simulink model "VCU_CS75_12_30_test"  (R2014a)
settings: Solver=FixedStepDiscrete  StartTime=0.0  StopTime=25  FixedStep=0.0005  RelTol=1e-3
InitFcn:
  | PID_canshu
values from neighbouring files (symbols this model uses):
  D1 = ecucoder_cal(D1)    [PID_canshu.m]
  D2 = ecucoder_cal(D2)    [PID_canshu.m]
  D3 = ecucoder_cal(D3)    [PID_canshu.m]
  ErrorLimit = ecucoder_cal(ErrorLimit)    [PID_canshu.m]
  ErrorSumMax1 = ecucoder_cal(ErrorSumMax1)    [PID_canshu.m]
  ErrorSumMax2 = ecucoder_cal(ErrorSumMax2)    [PID_canshu.m]
  ErrorSumMax3 = ecucoder_cal(ErrorSumMax3)    [PID_canshu.m]
  I1 = ecucoder_cal(I1)    [PID_canshu.m]
  I2 = ecucoder_cal(I2)    [PID_canshu.m]
  I3 = ecucoder_cal(I3)    [PID_canshu.m]
  Limit1 = ecucoder_cal(Limit1)    [PID_canshu.m]
  Limit2 = ecucoder_cal(Limit2)    [PID_canshu.m]
  P1 = ecucoder_cal(P1)    [PID_canshu.m]
  P2 = ecucoder_cal(P2)    [PID_canshu.m]
  P3 = ecucoder_cal(P3)    [PID_canshu.m]
  T_buchang = ecucoder_cal(T_buchang)    [PID_canshu.m]
undefined symbols (not defined in the file or in its folder): ecucoder_acal, I_SW01_L, LaterlAngleCommand, LDW, RemoteAcclPosition
libraries: simulink x940, ec5744lib x41
(part 10 of 31)

== system VCU_CS75_12_30_test/长安CS75底盘程序，20ms一次/Output/CAN0_Tx/to6003/C ==
  LongitudinalAcceleration_in : Inport
  LateralAcceleration_in : Inport  Port=2
  YawRate_in : Inport  Port=3
  C_DLC : Constant  Value=8  OutDataTypeStr=uint8
  C_DLC_Out : Terminator
  C_ID : Constant  Value=2147508227  OutDataTypeStr=single
  C_ID_Out : Terminator
  C_mux : Mux  Inputs=8
  Conv{1..8} (8 alike) : DataTypeConversion
  LateralAcceleration : Subsystem
  LongitudinalAcceleration : Subsystem
  YawRate : Subsystem
  or{1..8} (8 alike) : simulink/Logic and Bit Operations/Bitwise Operator  logicop=OR  UseBitMask=off  NumInputPorts=3  BitMask=bin2dec('11011001')  BitMaskRealWorld=Stored Integer
  output : Outport
  wires:
  C_mux/1 -> output/1
  LongitudinalAcceleration/1(output1) -> or1/1
  LongitudinalAcceleration/2(output2) -> or2/1
  LongitudinalAcceleration/3(output3) -> or3/1
  LongitudinalAcceleration/4(output4) -> or4/1
  LongitudinalAcceleration/5(output5) -> or5/1
  LongitudinalAcceleration/6(output6) -> or6/1
  LongitudinalAcceleration/7(output7) -> or7/1
  LongitudinalAcceleration/8(output8) -> or8/1
  LateralAcceleration/1(output1) -> or1/2
  LateralAcceleration/2(output2) -> or2/2
  LateralAcceleration/3(output3) -> or3/2
  LateralAcceleration/4(output4) -> or4/2
  LateralAcceleration/5(output5) -> or5/2
  LateralAcceleration/6(output6) -> or6/2
  LateralAcceleration/7(output7) -> or7/2
  LateralAcceleration/8(output8) -> or8/2
  YawRate/1(output1) -> or1/3
  YawRate/2(output2) -> or2/3
  YawRate/3(output3) -> or3/3
  YawRate/4(output4) -> or4/3
  YawRate/5(output5) -> or5/3
  YawRate/6(output6) -> or6/3
  YawRate/7(output7) -> or7/3
  YawRate/8(output8) -> or8/3
  or1/1 -> Conv1/1
  Conv1/1 -> C_mux/1
  or2/1 -> Conv2/1
  Conv2/1 -> C_mux/2
  or3/1 -> Conv3/1
  Conv3/1 -> C_mux/3
  or4/1 -> Conv4/1
  Conv4/1 -> C_mux/4
  or5/1 -> Conv5/1
  Conv5/1 -> C_mux/5
  or6/1 -> Conv6/1
  Conv6/1 -> C_mux/6
  or7/1 -> Conv7/1
  Conv7/1 -> C_mux/7
  or8/1 -> Conv8/1
  Conv8/1 -> C_mux/8
  C_ID/1 -> C_ID_Out/1
  C_DLC/1 -> C_DLC_Out/1
  LongitudinalAcceleration_in/1 -> LongitudinalAcceleration/1(LongitudinalAcceleration)
  LateralAcceleration_in/1 -> LateralAcceleration/1(LateralAcceleration)
  YawRate_in/1 -> YawRate/1(YawRate)

== system VCU_CS75_12_30_test/长安CS75底盘程序，20ms一次/Output/CAN0_Tx/to6004/D ==
  LongitudinalAutoDrivingState_in : Inport
  LateralAutoDrivingSwitch_in : Inport  Port=2
  FSM_CurrentState_in : Inport  Port=3
  ControllerErrorState_in : Inport  Port=4
  CommandSteering_in : Inport  Port=5
  Command_ACC_in : Inport  Port=6
  CommandSteering : Subsystem
  Command_ACC : Subsystem
  ControllerErrorState : Subsystem
  Conv{1..8} (8 alike) : DataTypeConversion
  D_DLC : Constant  Value=8  OutDataTypeStr=uint8
  D_DLC_Out : Terminator
  D_ID : Constant  Value=2147508228  OutDataTypeStr=single
  D_ID_Out : Terminator
  D_mux : Mux  Inputs=8
  FSM_CurrentState : Subsystem
  LateralAutoDrivingSwitch : Subsystem
  LongitudinalAutoDrivingState : Subsystem
  or{1..8} (8 alike) : simulink/Logic and Bit Operations/Bitwise Operator  logicop=OR  UseBitMask=off  NumInputPorts=6  BitMask=bin2dec('11011001')  BitMaskRealWorld=Stored Integer
  output : Outport
  wires:
  Command_ACC_in/1 -> Command_ACC/1(Command_ACC)
  CommandSteering_in/1 -> CommandSteering/1(CommandSteering)
  ControllerErrorState_in/1 -> ControllerErrorState/1(ControllerErrorState)
  FSM_CurrentState_in/1 -> FSM_CurrentState/1(FSM_CurrentState)
  LateralAutoDrivingSwitch_in/1 -> LateralAutoDrivingSwitch/1(LateralAutoDrivingSwitch)
  LongitudinalAutoDrivingState_in/1 -> LongitudinalAutoDrivingState/1(LongitudinalAutoDrivingState)
  D_DLC/1 -> D_DLC_Out/1
  D_ID/1 -> D_ID_Out/1
  Conv8/1 -> D_mux/8
  or8/1 -> Conv8/1
  Conv7/1 -> D_mux/7
  or7/1 -> Conv7/1
  Conv6/1 -> D_mux/6
  or6/1 -> Conv6/1
  Conv5/1 -> D_mux/5
  or5/1 -> Conv5/1
  Conv4/1 -> D_mux/4
  or4/1 -> Conv4/1
  Conv3/1 -> D_mux/3
  or3/1 -> Conv3/1
  Conv2/1 -> D_mux/2
  or2/1 -> Conv2/1
  Conv1/1 -> D_mux/1
  or1/1 -> Conv1/1
  Command_ACC/8(output8) -> or8/6
  Command_ACC/7(output7) -> or7/6
  Command_ACC/6(output6) -> or6/6
  Command_ACC/5(output5) -> or5/6
  Command_ACC/4(output4) -> or4/6
  Command_ACC/3(output3) -> or3/6
  Command_ACC/2(output2) -> or2/6
  Command_ACC/1(output1) -> or1/6
  CommandSteering/8(output8) -> or8/5
  CommandSteering/7(output7) -> or7/5
  CommandSteering/6(output6) -> or6/5
  CommandSteering/5(output5) -> or5/5
  CommandSteering/4(output4) -> or4/5
  CommandSteering/3(output3) -> or3/5
  CommandSteering/2(output2) -> or2/5
  CommandSteering/1(output1) -> or1/5
  ControllerErrorState/8(output8) -> or8/4
  ControllerErrorState/7(output7) -> or7/4
  ControllerErrorState/6(output6) -> or6/4
  ControllerErrorState/5(output5) -> or5/4
  ControllerErrorState/4(output4) -> or4/4
  ControllerErrorState/3(output3) -> or3/4
  ControllerErrorState/2(output2) -> or2/4
  ControllerErrorState/1(output1) -> or1/4
  FSM_CurrentState/8(output8) -> or8/3
  FSM_CurrentState/7(output7) -> or7/3
  FSM_CurrentState/6(output6) -> or6/3
  FSM_CurrentState/5(output5) -> or5/3
  FSM_CurrentState/4(output4) -> or4/3
  FSM_CurrentState/3(output3) -> or3/3
  FSM_CurrentState/2(output2) -> or2/3
  FSM_CurrentState/1(output1) -> or1/3
  LateralAutoDrivingSwitch/8(output8) -> or8/2
  LateralAutoDrivingSwitch/7(output7) -> or7/2
  LateralAutoDrivingSwitch/6(output6) -> or6/2
  LateralAutoDrivingSwitch/5(output5) -> or5/2
  LateralAutoDrivingSwitch/4(output4) -> or4/2
  LateralAutoDrivingSwitch/3(output3) -> or3/2
  LateralAutoDrivingSwitch/2(output2) -> or2/2
  LateralAutoDrivingSwitch/1(output1) -> or1/2
  LongitudinalAutoDrivingState/8(output8) -> or8/1
  LongitudinalAutoDrivingState/7(output7) -> or7/1
  LongitudinalAutoDrivingState/6(output6) -> or6/1
  LongitudinalAutoDrivingState/5(output5) -> or5/1
  LongitudinalAutoDrivingState/4(output4) -> or4/1
  LongitudinalAutoDrivingState/3(output3) -> or3/1
  LongitudinalAutoDrivingState/2(output2) -> or2/1
  LongitudinalAutoDrivingState/1(output1) -> or1/1
  D_mux/1 -> output/1

== system VCU_CS75_12_30_test/长安CS75底盘程序，20ms一次/Output/CAN0_Tx/to601/Message1 ==
  Error_in : Inport
  ErrorSum_in : Inport  Port=2
  PID_ST_Out_in : Inport  Port=3
  Conv{1..8} (8 alike) : DataTypeConversion
  Error : Subsystem
  ErrorSum : Subsystem
  Message601_DLC : Constant  Value=8  OutDataTypeStr=uint8
  Message601_DLC_Out : Terminator
  Message601_ID : Constant  Value=1537  OutDataTypeStr=single
  Message601_ID_Out : Terminator
  Message601_mux : Mux  Inputs=8
  PID_ST_Out : Subsystem
  or{1..8} (8 alike) : simulink/Logic and Bit Operations/Bitwise Operator  logicop=OR  UseBitMask=off  NumInputPorts=3  BitMask=bin2dec('11011001')  BitMaskRealWorld=Stored Integer
  output : Outport
  wires:
  PID_ST_Out_in/1 -> PID_ST_Out/1(PID_ST_Out)
  ErrorSum_in/1 -> ErrorSum/1(ErrorSum)
  Error_in/1 -> Error/1(Error)
  Message601_DLC/1 -> Message601_DLC_Out/1
  Message601_ID/1 -> Message601_ID_Out/1
  Conv8/1 -> Message601_mux/8
  or8/1 -> Conv8/1
  Conv7/1 -> Message601_mux/7
  or7/1 -> Conv7/1
  Conv6/1 -> Message601_mux/6
  or6/1 -> Conv6/1
  Conv5/1 -> Message601_mux/5
  or5/1 -> Conv5/1
  Conv4/1 -> Message601_mux/4
  or4/1 -> Conv4/1
  Conv3/1 -> Message601_mux/3
  or3/1 -> Conv3/1
  Conv2/1 -> Message601_mux/2
  or2/1 -> Conv2/1
  Conv1/1 -> Message601_mux/1
  or1/1 -> Conv1/1
  PID_ST_Out/8(output8) -> or8/3
  PID_ST_Out/7(output7) -> or7/3
  PID_ST_Out/6(output6) -> or6/3
  PID_ST_Out/5(output5) -> or5/3
  PID_ST_Out/4(output4) -> or4/3
  PID_ST_Out/3(output3) -> or3/3
  PID_ST_Out/2(output2) -> or2/3
  PID_ST_Out/1(output1) -> or1/3
  ErrorSum/8(output8) -> or8/2
  ErrorSum/7(output7) -> or7/2
  ErrorSum/6(output6) -> or6/2
  ErrorSum/5(output5) -> or5/2
  ErrorSum/4(output4) -> or4/2
  ErrorSum/3(output3) -> or3/2
  ErrorSum/2(output2) -> or2/2
  ErrorSum/1(output1) -> or1/2
  Error/8(output8) -> or8/1
  Error/7(output7) -> or7/1
  Error/6(output6) -> or6/1
  Error/5(output5) -> or5/1
  Error/4(output4) -> or4/1
  Error/3(output3) -> or3/1
  Error/2(output2) -> or2/1
  Error/1(output1) -> or1/1
  Message601_mux/1 -> output/1

== system VCU_CS75_12_30_test/长安CS75底盘程序，20ms一次/Output/CAN1_Tx/to28D/LAS_28D ==
  LAS_SLASpdLimitUnit_in : Inport
  LAS_LDWStatus_in : Inport  Port=2
  LAS_CaliStatus_in : Inport  Port=3
  LAS_TakeoverReq_in : Inport  Port=4
  LAS_DFDFailed_in : Inport  Port=5
  LAS_LDWVibrationWarning_in : Inport  Port=6
  LAS_SLASpdLimit_in : Inport  Port=7
  LAS_LDWReminder_in : Inport  Port=8
  LAS_DFDWarning_in : Inport  Port=9
  LAS_LASFailed_in : Inport  Port=10
  LAS_SteeringTorqueReq_in : Inport  Port=11
  LAS_SLAState_in : Inport  Port=12
  LAS_LKSStatus_in : Inport  Port=13
  RollingConter_in : Inport  Port=14
  CRC_in : Inport  Port=15
  CRC : Subsystem
  Conv{1..8} (8 alike) : DataTypeConversion
  LAS_28D_DLC : Constant  Value=8  OutDataTypeStr=uint8
  LAS_28D_DLC_Out : Terminator
  LAS_28D_ID : Constant  Value=653  OutDataTypeStr=single
  LAS_28D_ID_Out : Terminator
  LAS_28D_mux : Mux  Inputs=8
  LAS_CaliStatus : Subsystem
  LAS_DFDFailed : Subsystem
  LAS_DFDWarning : Subsystem
  LAS_LASFailed : Subsystem
  LAS_LDWReminder : Subsystem
  LAS_LDWStatus : Subsystem
  LAS_LDWVibrationWarning : Subsystem
  LAS_LKSStatus : Subsystem
  LAS_SLASpdLimit : Subsystem
  LAS_SLASpdLimitUnit : Subsystem
  LAS_SLAState : Subsystem
  LAS_SteeringTorqueReq : Subsystem
  LAS_TakeoverReq : Subsystem
  RollingConter : Subsystem
  or{1..8} (8 alike) : simulink/Logic and Bit Operations/Bitwise Operator  logicop=OR  UseBitMask=off  NumInputPorts=15  BitMask=bin2dec('11011001')  BitMaskRealWorld=Stored Integer
  output : Outport
  wires:
  LAS_28D_mux/1 -> output/1
  LAS_SLASpdLimitUnit/1(output1) -> or1/1
  LAS_SLASpdLimitUnit/2(output2) -> or2/1
  LAS_SLASpdLimitUnit/3(output3) -> or3/1
  LAS_SLASpdLimitUnit/4(output4) -> or4/1
  LAS_SLASpdLimitUnit/5(output5) -> or5/1
  LAS_SLASpdLimitUnit/6(output6) -> or6/1
  LAS_SLASpdLimitUnit/7(output7) -> or7/1
  LAS_SLASpdLimitUnit/8(output8) -> or8/1
  LAS_LDWStatus/1(output1) -> or1/2
  LAS_LDWStatus/2(output2) -> or2/2
  LAS_LDWStatus/3(output3) -> or3/2
  LAS_LDWStatus/4(output4) -> or4/2
  LAS_LDWStatus/5(output5) -> or5/2
  LAS_LDWStatus/6(output6) -> or6/2
  LAS_LDWStatus/7(output7) -> or7/2
  LAS_LDWStatus/8(output8) -> or8/2
  LAS_CaliStatus/1(output1) -> or1/3
  LAS_CaliStatus/2(output2) -> or2/3
  LAS_CaliStatus/3(output3) -> or3/3
  LAS_CaliStatus/4(output4) -> or4/3
  LAS_CaliStatus/5(output5) -> or5/3
  LAS_CaliStatus/6(output6) -> or6/3
  LAS_CaliStatus/7(output7) -> or7/3
  LAS_CaliStatus/8(output8) -> or8/3
  LAS_TakeoverReq/1(output1) -> or1/4
  LAS_TakeoverReq/2(output2) -> or2/4
  LAS_TakeoverReq/3(output3) -> or3/4
  LAS_TakeoverReq/4(output4) -> or4/4
  LAS_TakeoverReq/5(output5) -> or5/4
  LAS_TakeoverReq/6(output6) -> or6/4
  LAS_TakeoverReq/7(output7) -> or7/4
  LAS_TakeoverReq/8(output8) -> or8/4
  LAS_DFDFailed/1(output1) -> or1/5
  LAS_DFDFailed/2(output2) -> or2/5
  LAS_DFDFailed/3(output3) -> or3/5
  LAS_DFDFailed/4(output4) -> or4/5
  LAS_DFDFailed/5(output5) -> or5/5
  LAS_DFDFailed/6(output6) -> or6/5
  LAS_DFDFailed/7(output7) -> or7/5
  LAS_DFDFailed/8(output8) -> or8/5
  LAS_LDWVibrationWarning/1(output1) -> or1/6
  LAS_LDWVibrationWarning/2(output2) -> or2/6
  LAS_LDWVibrationWarning/3(output3) -> or3/6
  LAS_LDWVibrationWarning/4(output4) -> or4/6
  LAS_LDWVibrationWarning/5(output5) -> or5/6
  LAS_LDWVibrationWarning/6(output6) -> or6/6
  LAS_LDWVibrationWarning/7(output7) -> or7/6
  LAS_LDWVibrationWarning/8(output8) -> or8/6
  LAS_SLASpdLimit/1(output1) -> or1/7
  LAS_SLASpdLimit/2(output2) -> or2/7
  LAS_SLASpdLimit/3(output3) -> or3/7
  LAS_SLASpdLimit/4(output4) -> or4/7
  LAS_SLASpdLimit/5(output5) -> or5/7
  LAS_SLASpdLimit/6(output6) -> or6/7
  LAS_SLASpdLimit/7(output7) -> or7/7
  LAS_SLASpdLimit/8(output8) -> or8/7
  LAS_LDWReminder/1(output1) -> or1/8
  LAS_LDWReminder/2(output2) -> or2/8
  LAS_LDWReminder/3(output3) -> or3/8
  LAS_LDWReminder/4(output4) -> or4/8
  LAS_LDWReminder/5(output5) -> or5/8
  LAS_LDWReminder/6(output6) -> or6/8
  LAS_LDWReminder/7(output7) -> or7/8
  LAS_LDWReminder/8(output8) -> or8/8
  LAS_DFDWarning/1(output1) -> or1/9
  LAS_DFDWarning/2(output2) -> or2/9
  LAS_DFDWarning/3(output3) -> or3/9
  LAS_DFDWarning/4(output4) -> or4/9
  LAS_DFDWarning/5(output5) -> or5/9
  LAS_DFDWarning/6(output6) -> or6/9
  LAS_DFDWarning/7(output7) -> or7/9
  LAS_DFDWarning/8(output8) -> or8/9
  LAS_LASFailed/1(output1) -> or1/10
  LAS_LASFailed/2(output2) -> or2/10
  LAS_LASFailed/3(output3) -> or3/10
  LAS_LASFailed/4(output4) -> or4/10
  LAS_LASFailed/5(output5) -> or5/10
  LAS_LASFailed/6(output6) -> or6/10
  LAS_LASFailed/7(output7) -> or7/10
  LAS_LASFailed/8(output8) -> or8/10
  LAS_SteeringTorqueReq/1(output1) -> or1/11
  LAS_SteeringTorqueReq/2(output2) -> or2/11
  LAS_SteeringTorqueReq/3(output3) -> or3/11
  LAS_SteeringTorqueReq/4(output4) -> or4/11
  LAS_SteeringTorqueReq/5(output5) -> or5/11
  LAS_SteeringTorqueReq/6(output6) -> or6/11
  LAS_SteeringTorqueReq/7(output7) -> or7/11
  LAS_SteeringTorqueReq/8(output8) -> or8/11
  LAS_SLAState/1(output1) -> or1/12
  LAS_SLAState/2(output2) -> or2/12
  LAS_SLAState/3(output3) -> or3/12
  LAS_SLAState/4(output4) -> or4/12
  LAS_SLAState/5(output5) -> or5/12
  LAS_SLAState/6(output6) -> or6/12
  LAS_SLAState/7(output7) -> or7/12
  LAS_SLAState/8(output8) -> or8/12
  LAS_LKSStatus/1(output1) -> or1/13
  LAS_LKSStatus/2(output2) -> or2/13
  LAS_LKSStatus/3(output3) -> or3/13
  LAS_LKSStatus/4(output4) -> or4/13
  LAS_LKSStatus/5(output5) -> or5/13
  LAS_LKSStatus/6(output6) -> or6/13
  LAS_LKSStatus/7(output7) -> or7/13
  LAS_LKSStatus/8(output8) -> or8/13
  RollingConter/1(output1) -> or1/14
  RollingConter/2(output2) -> or2/14
  RollingConter/3(output3) -> or3/14
  RollingConter/4(output4) -> or4/14
  RollingConter/5(output5) -> or5/14
  RollingConter/6(output6) -> or6/14
  RollingConter/7(output7) -> or7/14
  RollingConter/8(output8) -> or8/14
  CRC/1(output1) -> or1/15
  CRC/2(output2) -> or2/15
  CRC/3(output3) -> or3/15
  CRC/4(output4) -> or4/15
  CRC/5(output5) -> or5/15
  CRC/6(output6) -> or6/15
  CRC/7(output7) -> or7/15
  CRC/8(output8) -> or8/15
  or1/1 -> Conv1/1
  Conv1/1 -> LAS_28D_mux/1
  or2/1 -> Conv2/1
  Conv2/1 -> LAS_28D_mux/2
  or3/1 -> Conv3/1
  Conv3/1 -> LAS_28D_mux/3
  or4/1 -> Conv4/1
  Conv4/1 -> LAS_28D_mux/4
  or5/1 -> Conv5/1
  Conv5/1 -> LAS_28D_mux/5
  or6/1 -> Conv6/1
  Conv6/1 -> LAS_28D_mux/6
  or7/1 -> Conv7/1
  Conv7/1 -> LAS_28D_mux/7
  or8/1 -> Conv8/1
  Conv8/1 -> LAS_28D_mux/8
  LAS_28D_ID/1 -> LAS_28D_ID_Out/1
  LAS_28D_DLC/1 -> LAS_28D_DLC_Out/1
  LAS_SLASpdLimitUnit_in/1 -> LAS_SLASpdLimitUnit/1(LAS_SLASpdLimitUnit)
  LAS_LDWStatus_in/1 -> LAS_LDWStatus/1(LAS_LDWStatus)
  LAS_CaliStatus_in/1 -> LAS_CaliStatus/1(LAS_CaliStatus)
  LAS_TakeoverReq_in/1 -> LAS_TakeoverReq/1(LAS_TakeoverReq)
  LAS_DFDFailed_in/1 -> LAS_DFDFailed/1(LAS_DFDFailed)
  LAS_LDWVibrationWarning_in/1 -> LAS_LDWVibrationWarning/1(LAS_LDWVibrationWarning)
  LAS_SLASpdLimit_in/1 -> LAS_SLASpdLimit/1(LAS_SLASpdLimit)
  LAS_LDWReminder_in/1 -> LAS_LDWReminder/1(LAS_LDWReminder)
  LAS_DFDWarning_in/1 -> LAS_DFDWarning/1(LAS_DFDWarning)
  LAS_LASFailed_in/1 -> LAS_LASFailed/1(LAS_LASFailed)
  LAS_SteeringTorqueReq_in/1 -> LAS_SteeringTorqueReq/1(LAS_SteeringTorqueReq)
  LAS_SLAState_in/1 -> LAS_SLAState/1(LAS_SLAState)
  LAS_LKSStatus_in/1 -> LAS_LKSStatus/1(LAS_LKSStatus)
  RollingConter_in/1 -> RollingConter/1(RollingConter)
  CRC_in/1 -> CRC/1(CRC)

== system VCU_CS75_12_30_test/长安CS75底盘程序，20ms一次/Output/CAN1_Tx/to2E4/ACC_2E4 ==
  ACC_CDDAxEnable_in : Inport
  ACC_DecToStop_in : Inport  Port=2
  ACC_Driveoff_Request_in : Inport  Port=3
  ACC_Mode_in : Inport  Port=4
  ACC_ACCTargetAcceleration_in : Inport  Port=5
  ACC_RollingCounter_id_in : Inport  Port=6
  ACC_CheckSum_id_in : Inport  Port=7
  ACC_2E4_DLC : Constant  Value=8  OutDataTypeStr=uint8
  ACC_2E4_DLC_Out : Terminator
  ACC_2E4_ID : Constant  Value=740  OutDataTypeStr=single
  ACC_2E4_ID_Out : Terminator
  ACC_2E4_mux : Mux  Inputs=8
  ACC_ACCTargetAcceleration : Subsystem
  ACC_CDDAxEnable : Subsystem
  ACC_CheckSum_id : Subsystem
  ACC_DecToStop : Subsystem
  ACC_Driveoff_Request : Subsystem
  ACC_Mode : Subsystem
  ACC_RollingCounter_id : Subsystem
  Conv{1..8} (8 alike) : DataTypeConversion
  or{1..8} (8 alike) : simulink/Logic and Bit Operations/Bitwise Operator  logicop=OR  UseBitMask=off  NumInputPorts=7  BitMask=bin2dec('11011001')  BitMaskRealWorld=Stored Integer
  output : Outport
  wires:
  ACC_2E4_mux/1 -> output/1
  ACC_CDDAxEnable/1(output1) -> or1/1
  ACC_CDDAxEnable/2(output2) -> or2/1
  ACC_CDDAxEnable/3(output3) -> or3/1
  ACC_CDDAxEnable/4(output4) -> or4/1
  ACC_CDDAxEnable/5(output5) -> or5/1
  ACC_CDDAxEnable/6(output6) -> or6/1
  ACC_CDDAxEnable/7(output7) -> or7/1
  ACC_CDDAxEnable/8(output8) -> or8/1
  ACC_DecToStop/1(output1) -> or1/2
  ACC_DecToStop/2(output2) -> or2/2
  ACC_DecToStop/3(output3) -> or3/2
  ACC_DecToStop/4(output4) -> or4/2
  ACC_DecToStop/5(output5) -> or5/2
  ACC_DecToStop/6(output6) -> or6/2
  ACC_DecToStop/7(output7) -> or7/2
  ACC_DecToStop/8(output8) -> or8/2
  ACC_Driveoff_Request/1(output1) -> or1/3
  ACC_Driveoff_Request/2(output2) -> or2/3
  ACC_Driveoff_Request/3(output3) -> or3/3
  ACC_Driveoff_Request/4(output4) -> or4/3
  ACC_Driveoff_Request/5(output5) -> or5/3
  ACC_Driveoff_Request/6(output6) -> or6/3
  ACC_Driveoff_Request/7(output7) -> or7/3
  ACC_Driveoff_Request/8(output8) -> or8/3
  ACC_Mode/1(output1) -> or1/4
  ACC_Mode/2(output2) -> or2/4
  ACC_Mode/3(output3) -> or3/4
  ACC_Mode/4(output4) -> or4/4
  ACC_Mode/5(output5) -> or5/4
  ACC_Mode/6(output6) -> or6/4
  ACC_Mode/7(output7) -> or7/4
  ACC_Mode/8(output8) -> or8/4
  ACC_ACCTargetAcceleration/1(output1) -> or1/5
  ACC_ACCTargetAcceleration/2(output2) -> or2/5
  ACC_ACCTargetAcceleration/3(output3) -> or3/5
  ACC_ACCTargetAcceleration/4(output4) -> or4/5
  ACC_ACCTargetAcceleration/5(output5) -> or5/5
  ACC_ACCTargetAcceleration/6(output6) -> or6/5
  ACC_ACCTargetAcceleration/7(output7) -> or7/5
  ACC_ACCTargetAcceleration/8(output8) -> or8/5
  ACC_RollingCounter_id/1(output1) -> or1/6
  ACC_RollingCounter_id/2(output2) -> or2/6
  ACC_RollingCounter_id/3(output3) -> or3/6
  ACC_RollingCounter_id/4(output4) -> or4/6
  ACC_RollingCounter_id/5(output5) -> or5/6
  ACC_RollingCounter_id/6(output6) -> or6/6
  ACC_RollingCounter_id/7(output7) -> or7/6
  ACC_RollingCounter_id/8(output8) -> or8/6
  ACC_CheckSum_id/1(output1) -> or1/7
  ACC_CheckSum_id/2(output2) -> or2/7
  ACC_CheckSum_id/3(output3) -> or3/7
  ACC_CheckSum_id/4(output4) -> or4/7
  ACC_CheckSum_id/5(output5) -> or5/7
  ACC_CheckSum_id/6(output6) -> or6/7
  ACC_CheckSum_id/7(output7) -> or7/7
  ACC_CheckSum_id/8(output8) -> or8/7
  or1/1 -> Conv1/1
  Conv1/1 -> ACC_2E4_mux/1
  or2/1 -> Conv2/1
  Conv2/1 -> ACC_2E4_mux/2
  or3/1 -> Conv3/1
  Conv3/1 -> ACC_2E4_mux/3
  or4/1 -> Conv4/1
  Conv4/1 -> ACC_2E4_mux/4
  or5/1 -> Conv5/1
  Conv5/1 -> ACC_2E4_mux/5
  or6/1 -> Conv6/1
  Conv6/1 -> ACC_2E4_mux/6
  or7/1 -> Conv7/1
  Conv7/1 -> ACC_2E4_mux/7
  or8/1 -> Conv8/1
  Conv8/1 -> ACC_2E4_mux/8
  ACC_2E4_ID/1 -> ACC_2E4_ID_Out/1
  ACC_2E4_DLC/1 -> ACC_2E4_DLC_Out/1
  ACC_CDDAxEnable_in/1 -> ACC_CDDAxEnable/1(ACC_CDDAxEnable)
  ACC_DecToStop_in/1 -> ACC_DecToStop/1(ACC_DecToStop)
  ACC_Driveoff_Request_in/1 -> ACC_Driveoff_Request/1(ACC_Driveoff_Request)
  ACC_Mode_in/1 -> ACC_Mode/1(ACC_Mode)
  ACC_ACCTargetAcceleration_in/1 -> ACC_ACCTargetAcceleration/1(ACC_ACCTargetAcceleration)
  ACC_RollingCounter_id_in/1 -> ACC_RollingCounter_id/1(ACC_RollingCounter_id)
  ACC_CheckSum_id_in/1 -> ACC_CheckSum_id/1(ACC_CheckSum_id)

== system VCU_CS75_12_30_test/长安CS75底盘程序，20ms一次/Output/CAN1_Tx/to2E5/ACC_2E5 ==
  ACC_AEBTargetDeceleration_in : Inport
  ACC_AccTrqReqEnable_in : Inport  Port=2
  ACC_AWBlevel_in : Inport  Port=3
  ACC_ABAavailable_in : Inport  Port=4
  ACC_AEBLVehilcehold_in : Inport  Port=5
  ACC_PCWPreWarning_in : Inport  Port=6
  ACC_PCW_LatentWarning_in : Inport  Port=7
  ACC_PCWPenable_in : Inport  Port=8
  ACC_ESPPrefill_in : Inport  Port=9
  ACC_AWBavailable_in : Inport  Port=10
  ACC_AccTorqueReq_in : Inport  Port=11
  ACC_ABAlevel_in : Inport  Port=12
  ACC_AEBDecCtrlAvail_in : Inport  Port=13
  ACC_TextInfoForDriver_in : Inport  Port=14
  ACC_RollingCounter_in : Inport  Port=15
  ACC_CheckSum_in : Inport  Port=16
  ACC_2E5_DLC : Constant  Value=8  OutDataTypeStr=uint8
  ACC_2E5_DLC_Out : Terminator
  ACC_2E5_ID : Constant  Value=741  OutDataTypeStr=single
  ACC_2E5_ID_Out : Terminator
  ACC_2E5_mux : Mux  Inputs=8
  ACC_ABAavailable : Subsystem
  ACC_ABAlevel : Subsystem
  ACC_AEBDecCtrlAvail : Subsystem
  ACC_AEBLVehilcehold : Subsystem
  ACC_AEBTargetDeceleration : Subsystem
  ACC_AWBavailable : Subsystem
  ACC_AWBlevel : Subsystem
  ACC_AccTorqueReq : Subsystem
  ACC_AccTrqReqEnable : Subsystem
  ACC_CheckSum : Subsystem
  ACC_ESPPrefill : Subsystem
  ACC_PCWPenable : Subsystem
  ACC_PCWPreWarning : Subsystem
  ACC_PCW_LatentWarning : Subsystem
  ACC_RollingCounter : Subsystem
  ACC_TextInfoForDriver : Subsystem
  Conv{1..8} (8 alike) : DataTypeConversion
  or{1..8} (8 alike) : simulink/Logic and Bit Operations/Bitwise Operator  logicop=OR  UseBitMask=off  NumInputPorts=16  BitMask=bin2dec('11011001')  BitMaskRealWorld=Stored Integer
  output : Outport
  wires:
  ACC_2E5_mux/1 -> output/1
  ACC_AEBTargetDeceleration/1(output1) -> or1/1
  ACC_AEBTargetDeceleration/2(output2) -> or2/1
  ACC_AEBTargetDeceleration/3(output3) -> or3/1
  ACC_AEBTargetDeceleration/4(output4) -> or4/1
  ACC_AEBTargetDeceleration/5(output5) -> or5/1
  ACC_AEBTargetDeceleration/6(output6) -> or6/1
  ACC_AEBTargetDeceleration/7(output7) -> or7/1
  ACC_AEBTargetDeceleration/8(output8) -> or8/1
  ACC_AccTrqReqEnable/1(output1) -> or1/2
  ACC_AccTrqReqEnable/2(output2) -> or2/2
  ACC_AccTrqReqEnable/3(output3) -> or3/2
  ACC_AccTrqReqEnable/4(output4) -> or4/2
  ACC_AccTrqReqEnable/5(output5) -> or5/2
  ACC_AccTrqReqEnable/6(output6) -> or6/2
  ACC_AccTrqReqEnable/7(output7) -> or7/2
  ACC_AccTrqReqEnable/8(output8) -> or8/2
  ACC_AWBlevel/1(output1) -> or1/3
  ACC_AWBlevel/2(output2) -> or2/3
  ACC_AWBlevel/3(output3) -> or3/3
  ACC_AWBlevel/4(output4) -> or4/3
  ACC_AWBlevel/5(output5) -> or5/3
  ACC_AWBlevel/6(output6) -> or6/3
  ACC_AWBlevel/7(output7) -> or7/3
  ACC_AWBlevel/8(output8) -> or8/3
  ACC_ABAavailable/1(output1) -> or1/4
  ACC_ABAavailable/2(output2) -> or2/4
  ACC_ABAavailable/3(output3) -> or3/4
  ACC_ABAavailable/4(output4) -> or4/4
  ACC_ABAavailable/5(output5) -> or5/4
  ACC_ABAavailable/6(output6) -> or6/4
  ACC_ABAavailable/7(output7) -> or7/4
  ACC_ABAavailable/8(output8) -> or8/4
  ACC_AEBLVehilcehold/1(output1) -> or1/5
  ACC_AEBLVehilcehold/2(output2) -> or2/5
  ACC_AEBLVehilcehold/3(output3) -> or3/5
  ACC_AEBLVehilcehold/4(output4) -> or4/5
  ACC_AEBLVehilcehold/5(output5) -> or5/5
  ACC_AEBLVehilcehold/6(output6) -> or6/5
  ACC_AEBLVehilcehold/7(output7) -> or7/5
  ACC_AEBLVehilcehold/8(output8) -> or8/5
  ACC_PCWPreWarning/1(output1) -> or1/6
  ACC_PCWPreWarning/2(output2) -> or2/6
  ACC_PCWPreWarning/3(output3) -> or3/6
  ACC_PCWPreWarning/4(output4) -> or4/6
  ACC_PCWPreWarning/5(output5) -> or5/6
  ACC_PCWPreWarning/6(output6) -> or6/6
  ACC_PCWPreWarning/7(output7) -> or7/6
  ACC_PCWPreWarning/8(output8) -> or8/6
  ACC_PCW_LatentWarning/1(output1) -> or1/7
  ACC_PCW_LatentWarning/2(output2) -> or2/7
  ACC_PCW_LatentWarning/3(output3) -> or3/7
  ACC_PCW_LatentWarning/4(output4) -> or4/7
  ACC_PCW_LatentWarning/5(output5) -> or5/7
  ACC_PCW_LatentWarning/6(output6) -> or6/7
  ACC_PCW_LatentWarning/7(output7) -> or7/7
  ACC_PCW_LatentWarning/8(output8) -> or8/7
  ACC_PCWPenable/1(output1) -> or1/8
  ACC_PCWPenable/2(output2) -> or2/8
  ACC_PCWPenable/3(output3) -> or3/8
  ACC_PCWPenable/4(output4) -> or4/8
  ACC_PCWPenable/5(output5) -> or5/8
  ACC_PCWPenable/6(output6) -> or6/8
  ACC_PCWPenable/7(output7) -> or7/8
  ACC_PCWPenable/8(output8) -> or8/8
  ACC_ESPPrefill/1(output1) -> or1/9
  ACC_ESPPrefill/2(output2) -> or2/9
  ACC_ESPPrefill/3(output3) -> or3/9
  ACC_ESPPrefill/4(output4) -> or4/9
  ACC_ESPPrefill/5(output5) -> or5/9
  ACC_ESPPrefill/6(output6) -> or6/9
  ACC_ESPPrefill/7(output7) -> or7/9
  ACC_ESPPrefill/8(output8) -> or8/9
  ACC_AWBavailable/1(output1) -> or1/10
  ACC_AWBavailable/2(output2) -> or2/10
  ACC_AWBavailable/3(output3) -> or3/10
  ACC_AWBavailable/4(output4) -> or4/10
  ACC_AWBavailable/5(output5) -> or5/10
  ACC_AWBavailable/6(output6) -> or6/10
  ACC_AWBavailable/7(output7) -> or7/10
  ACC_AWBavailable/8(output8) -> or8/10
  ACC_AccTorqueReq/1(output1) -> or1/11
  ACC_AccTorqueReq/2(output2) -> or2/11
  ACC_AccTorqueReq/3(output3) -> or3/11
  ACC_AccTorqueReq/4(output4) -> or4/11
  ACC_AccTorqueReq/5(output5) -> or5/11
  ACC_AccTorqueReq/6(output6) -> or6/11
  ACC_AccTorqueReq/7(output7) -> or7/11
  ACC_AccTorqueReq/8(output8) -> or8/11
  ACC_ABAlevel/1(output1) -> or1/12
  ACC_ABAlevel/2(output2) -> or2/12
  ACC_ABAlevel/3(output3) -> or3/12
  ACC_ABAlevel/4(output4) -> or4/12
  ACC_ABAlevel/5(output5) -> or5/12
  ACC_ABAlevel/6(output6) -> or6/12
  ACC_ABAlevel/7(output7) -> or7/12
  ACC_ABAlevel/8(output8) -> or8/12
  ACC_AEBDecCtrlAvail/1(output1) -> or1/13
  ACC_AEBDecCtrlAvail/2(output2) -> or2/13
  ACC_AEBDecCtrlAvail/3(output3) -> or3/13
  ACC_AEBDecCtrlAvail/4(output4) -> or4/13
  ACC_AEBDecCtrlAvail/5(output5) -> or5/13
  ACC_AEBDecCtrlAvail/6(output6) -> or6/13
  ACC_AEBDecCtrlAvail/7(output7) -> or7/13
  ACC_AEBDecCtrlAvail/8(output8) -> or8/13
  ACC_TextInfoForDriver/1(output1) -> or1/14
  ACC_TextInfoForDriver/2(output2) -> or2/14
  ACC_TextInfoForDriver/3(output3) -> or3/14
  ACC_TextInfoForDriver/4(output4) -> or4/14
  ACC_TextInfoForDriver/5(output5) -> or5/14
  ACC_TextInfoForDriver/6(output6) -> or6/14
  ACC_TextInfoForDriver/7(output7) -> or7/14
  ACC_TextInfoForDriver/8(output8) -> or8/14
  ACC_RollingCounter/1(output1) -> or1/15
  ACC_RollingCounter/2(output2) -> or2/15
  ACC_RollingCounter/3(output3) -> or3/15
  ACC_RollingCounter/4(output4) -> or4/15
  ACC_RollingCounter/5(output5) -> or5/15
  ACC_RollingCounter/6(output6) -> or6/15
  ACC_RollingCounter/7(output7) -> or7/15
  ACC_RollingCounter/8(output8) -> or8/15
  ACC_CheckSum/1(output1) -> or1/16
  ACC_CheckSum/2(output2) -> or2/16
  ACC_CheckSum/3(output3) -> or3/16
  ACC_CheckSum/4(output4) -> or4/16
  ACC_CheckSum/5(output5) -> or5/16
  ACC_CheckSum/6(output6) -> or6/16
  ACC_CheckSum/7(output7) -> or7/16
  ACC_CheckSum/8(output8) -> or8/16
  or1/1 -> Conv1/1
  Conv1/1 -> ACC_2E5_mux/1
  or2/1 -> Conv2/1
  Conv2/1 -> ACC_2E5_mux/2
  or3/1 -> Conv3/1
  Conv3/1 -> ACC_2E5_mux/3
  or4/1 -> Conv4/1
  Conv4/1 -> ACC_2E5_mux/4
  or5/1 -> Conv5/1
  Conv5/1 -> ACC_2E5_mux/5
  or6/1 -> Conv6/1
  Conv6/1 -> ACC_2E5_mux/6
  or7/1 -> Conv7/1
  Conv7/1 -> ACC_2E5_mux/7
  or8/1 -> Conv8/1
  Conv8/1 -> ACC_2E5_mux/8
  ACC_2E5_ID/1 -> ACC_2E5_ID_Out/1
  ACC_2E5_DLC/1 -> ACC_2E5_DLC_Out/1
  ACC_AEBTargetDeceleration_in/1 -> ACC_AEBTargetDeceleration/1(ACC_AEBTargetDeceleration)
  ACC_AccTrqReqEnable_in/1 -> ACC_AccTrqReqEnable/1(ACC_AccTrqReqEnable)
  ACC_AWBlevel_in/1 -> ACC_AWBlevel/1(ACC_AWBlevel)
  ACC_ABAavailable_in/1 -> ACC_ABAavailable/1(ACC_ABAavailable)
  ACC_AEBLVehilcehold_in/1 -> ACC_AEBLVehilcehold/1(ACC_AEBLVehilcehold)
  ACC_PCWPreWarning_in/1 -> ACC_PCWPreWarning/1(ACC_PCWPreWarning)
  ACC_PCW_LatentWarning_in/1 -> ACC_PCW_LatentWarning/1(ACC_PCW_LatentWarning)
  ACC_PCWPenable_in/1 -> ACC_PCWPenable/1(ACC_PCWPenable)
  ACC_ESPPrefill_in/1 -> ACC_ESPPrefill/1(ACC_ESPPrefill)
  ACC_AWBavailable_in/1 -> ACC_AWBavailable/1(ACC_AWBavailable)
  ACC_AccTorqueReq_in/1 -> ACC_AccTorqueReq/1(ACC_AccTorqueReq)
  ACC_ABAlevel_in/1 -> ACC_ABAlevel/1(ACC_ABAlevel)
  ACC_AEBDecCtrlAvail_in/1 -> ACC_AEBDecCtrlAvail/1(ACC_AEBDecCtrlAvail)
  ACC_TextInfoForDriver_in/1 -> ACC_TextInfoForDriver/1(ACC_TextInfoForDriver)
  ACC_RollingCounter_in/1 -> ACC_RollingCounter/1(ACC_RollingCounter)
  ACC_CheckSum_in/1 -> ACC_CheckSum/1(ACC_CheckSum)

== system VCU_CS75_12_30_test/长安CS75底盘程序，20ms一次/Output/Subsystem/28A/APA_28A ==
  APA_SteeringAngleReqProtection_in : Inport
  APA_EPSAngleReq_in : Inport  Port=2
  APA_Indication_in : Inport  Port=3
  APA_OnOff_in : Inport  Port=4
  APA_IncreasePressureReq_in : Inport  Port=5
  APA_RollingCounter_in : Inport  Port=6
  APA_CheckSum_in : Inport  Port=7
  APA_28A_DLC : Constant  Value=8  OutDataTypeStr=uint8
  APA_28A_DLC_Out : Terminator
  APA_28A_ID : Constant  Value=650  OutDataTypeStr=single
  APA_28A_ID_Out : Terminator
  APA_28A_mux : Mux  Inputs=8
  APA_CheckSum : Subsystem
  APA_EPSAngleReq : Subsystem
  APA_IncreasePressureReq : Subsystem
  APA_Indication : Subsystem
  APA_OnOff : Subsystem
  APA_RollingCounter : Subsystem
  APA_SteeringAngleReqProtection : Subsystem
  Conv{1..8} (8 alike) : DataTypeConversion
  or{1..8} (8 alike) : simulink/Logic and Bit Operations/Bitwise Operator  logicop=OR  UseBitMask=off  NumInputPorts=7  BitMask=bin2dec('11011001')  BitMaskRealWorld=Stored Integer
  output : Outport
  wires:
  APA_CheckSum_in/1 -> APA_CheckSum/1(APA_CheckSum)
  APA_RollingCounter_in/1 -> APA_RollingCounter/1(APA_RollingCounter)
  APA_IncreasePressureReq_in/1 -> APA_IncreasePressureReq/1(APA_IncreasePressureReq)
  APA_OnOff_in/1 -> APA_OnOff/1(APA_OnOff)
  APA_Indication_in/1 -> APA_Indication/1(APA_Indication)
  APA_EPSAngleReq_in/1 -> APA_EPSAngleReq/1(APA_EPSAngleReq)
  APA_SteeringAngleReqProtection_in/1 -> APA_SteeringAngleReqProtection/1(APA_SteeringAngleReqProtection)
  APA_28A_DLC/1 -> APA_28A_DLC_Out/1
  APA_28A_ID/1 -> APA_28A_ID_Out/1
  Conv8/1 -> APA_28A_mux/8
  or8/1 -> Conv8/1
  Conv7/1 -> APA_28A_mux/7
  or7/1 -> Conv7/1
  Conv6/1 -> APA_28A_mux/6
  or6/1 -> Conv6/1
  Conv5/1 -> APA_28A_mux/5
  or5/1 -> Conv5/1
  Conv4/1 -> APA_28A_mux/4
  or4/1 -> Conv4/1
  Conv3/1 -> APA_28A_mux/3
  or3/1 -> Conv3/1
  Conv2/1 -> APA_28A_mux/2
  or2/1 -> Conv2/1
  Conv1/1 -> APA_28A_mux/1
  or1/1 -> Conv1/1
  APA_CheckSum/8(output8) -> or8/7
  APA_CheckSum/7(output7) -> or7/7
  APA_CheckSum/6(output6) -> or6/7
  APA_CheckSum/5(output5) -> or5/7
  APA_CheckSum/4(output4) -> or4/7
  APA_CheckSum/3(output3) -> or3/7
  APA_CheckSum/2(output2) -> or2/7
  APA_CheckSum/1(output1) -> or1/7
  APA_RollingCounter/8(output8) -> or8/6
  APA_RollingCounter/7(output7) -> or7/6
  APA_RollingCounter/6(output6) -> or6/6
  APA_RollingCounter/5(output5) -> or5/6
  APA_RollingCounter/4(output4) -> or4/6
  APA_RollingCounter/3(output3) -> or3/6
  APA_RollingCounter/2(output2) -> or2/6
  APA_RollingCounter/1(output1) -> or1/6
  APA_IncreasePressureReq/8(output8) -> or8/5
  APA_IncreasePressureReq/7(output7) -> or7/5
  APA_IncreasePressureReq/6(output6) -> or6/5
  APA_IncreasePressureReq/5(output5) -> or5/5
  APA_IncreasePressureReq/4(output4) -> or4/5
  APA_IncreasePressureReq/3(output3) -> or3/5
  APA_IncreasePressureReq/2(output2) -> or2/5
  APA_IncreasePressureReq/1(output1) -> or1/5
  APA_OnOff/8(output8) -> or8/4
  APA_OnOff/7(output7) -> or7/4
  APA_OnOff/6(output6) -> or6/4
  APA_OnOff/5(output5) -> or5/4
  APA_OnOff/4(output4) -> or4/4
  APA_OnOff/3(output3) -> or3/4
  APA_OnOff/2(output2) -> or2/4
  APA_OnOff/1(output1) -> or1/4
  APA_Indication/8(output8) -> or8/3
  APA_Indication/7(output7) -> or7/3
  APA_Indication/6(output6) -> or6/3
  APA_Indication/5(output5) -> or5/3
  APA_Indication/4(output4) -> or4/3
  APA_Indication/3(output3) -> or3/3
  APA_Indication/2(output2) -> or2/3
  APA_Indication/1(output1) -> or1/3
  APA_EPSAngleReq/8(output8) -> or8/2
  APA_EPSAngleReq/7(output7) -> or7/2
  APA_EPSAngleReq/6(output6) -> or6/2
  APA_EPSAngleReq/5(output5) -> or5/2
  APA_EPSAngleReq/4(output4) -> or4/2
  APA_EPSAngleReq/3(output3) -> or3/2
  APA_EPSAngleReq/2(output2) -> or2/2
  APA_EPSAngleReq/1(output1) -> or1/2
  APA_SteeringAngleReqProtection/8(output8) -> or8/1
  APA_SteeringAngleReqProtection/7(output7) -> or7/1
  APA_SteeringAngleReqProtection/6(output6) -> or6/1
  APA_SteeringAngleReqProtection/5(output5) -> or5/1
  APA_SteeringAngleReqProtection/4(output4) -> or4/1
  APA_SteeringAngleReqProtection/3(output3) -> or3/1
  APA_SteeringAngleReqProtection/2(output2) -> or2/1
  APA_SteeringAngleReqProtection/1(output1) -> or1/1
  APA_28A_mux/1 -> output/1

== system VCU_CS75_12_30_test/长安CS75底盘程序，20ms一次/Output/Subsystem/28D/LAS_28D ==
  LAS_SLASpdLimitUnit_in : Inport
  LAS_LDWStatus_in : Inport  Port=2
  LAS_CaliStatus_in : Inport  Port=3
  LAS_TakeoverReq_in : Inport  Port=4
  LAS_DFDFailed_in : Inport  Port=5
  LAS_LDWVibrationWarning_in : Inport  Port=6
  LAS_SLASpdLimit_in : Inport  Port=7
  LAS_LDWReminder_in : Inport  Port=8
  LAS_DFDWarning_in : Inport  Port=9
  LAS_LASFailed_in : Inport  Port=10
  LAS_SteeringTorqueReq_in : Inport  Port=11
  LAS_SLAState_in : Inport  Port=12
  LAS_LKSStatus_in : Inport  Port=13
  RollingConter_in : Inport  Port=14
  CRC_in : Inport  Port=15
  CRC : Subsystem
  Conv{1..8} (8 alike) : DataTypeConversion
  LAS_28D_DLC : Constant  Value=8  OutDataTypeStr=uint8
  LAS_28D_DLC_Out : Terminator
  LAS_28D_ID : Constant  Value=653  OutDataTypeStr=single
  LAS_28D_ID_Out : Terminator
  LAS_28D_mux : Mux  Inputs=8
  LAS_CaliStatus : Subsystem
  LAS_DFDFailed : Subsystem
  LAS_DFDWarning : Subsystem
  LAS_LASFailed : Subsystem
  LAS_LDWReminder : Subsystem
  LAS_LDWStatus : Subsystem
  LAS_LDWVibrationWarning : Subsystem
  LAS_LKSStatus : Subsystem
  LAS_SLASpdLimit : Subsystem
  LAS_SLASpdLimitUnit : Subsystem
  LAS_SLAState : Subsystem
  LAS_SteeringTorqueReq : Subsystem
  LAS_TakeoverReq : Subsystem
  RollingConter : Subsystem
  or{1..8} (8 alike) : simulink/Logic and Bit Operations/Bitwise Operator  logicop=OR  UseBitMask=off  NumInputPorts=15  BitMask=bin2dec('11011001')  BitMaskRealWorld=Stored Integer
  output : Outport
  wires:
  LAS_28D_mux/1 -> output/1
  LAS_SLASpdLimitUnit/1(output1) -> or1/1
  LAS_SLASpdLimitUnit/2(output2) -> or2/1
  LAS_SLASpdLimitUnit/3(output3) -> or3/1
  LAS_SLASpdLimitUnit/4(output4) -> or4/1
  LAS_SLASpdLimitUnit/5(output5) -> or5/1
  LAS_SLASpdLimitUnit/6(output6) -> or6/1
  LAS_SLASpdLimitUnit/7(output7) -> or7/1
  LAS_SLASpdLimitUnit/8(output8) -> or8/1
  LAS_LDWStatus/1(output1) -> or1/2
  LAS_LDWStatus/2(output2) -> or2/2
  LAS_LDWStatus/3(output3) -> or3/2
  LAS_LDWStatus/4(output4) -> or4/2
  LAS_LDWStatus/5(output5) -> or5/2
  LAS_LDWStatus/6(output6) -> or6/2
  LAS_LDWStatus/7(output7) -> or7/2
  LAS_LDWStatus/8(output8) -> or8/2
  LAS_CaliStatus/1(output1) -> or1/3
  LAS_CaliStatus/2(output2) -> or2/3
  LAS_CaliStatus/3(output3) -> or3/3
  LAS_CaliStatus/4(output4) -> or4/3
  LAS_CaliStatus/5(output5) -> or5/3
  LAS_CaliStatus/6(output6) -> or6/3
  LAS_CaliStatus/7(output7) -> or7/3
  LAS_CaliStatus/8(output8) -> or8/3
  LAS_TakeoverReq/1(output1) -> or1/4
  LAS_TakeoverReq/2(output2) -> or2/4
  LAS_TakeoverReq/3(output3) -> or3/4
  LAS_TakeoverReq/4(output4) -> or4/4
  LAS_TakeoverReq/5(output5) -> or5/4
  LAS_TakeoverReq/6(output6) -> or6/4
  LAS_TakeoverReq/7(output7) -> or7/4
  LAS_TakeoverReq/8(output8) -> or8/4
  LAS_DFDFailed/1(output1) -> or1/5
  LAS_DFDFailed/2(output2) -> or2/5
  LAS_DFDFailed/3(output3) -> or3/5
  LAS_DFDFailed/4(output4) -> or4/5
  LAS_DFDFailed/5(output5) -> or5/5
  LAS_DFDFailed/6(output6) -> or6/5
  LAS_DFDFailed/7(output7) -> or7/5
  LAS_DFDFailed/8(output8) -> or8/5
  LAS_LDWVibrationWarning/1(output1) -> or1/6
  LAS_LDWVibrationWarning/2(output2) -> or2/6
  LAS_LDWVibrationWarning/3(output3) -> or3/6
  LAS_LDWVibrationWarning/4(output4) -> or4/6
  LAS_LDWVibrationWarning/5(output5) -> or5/6
  LAS_LDWVibrationWarning/6(output6) -> or6/6
  LAS_LDWVibrationWarning/7(output7) -> or7/6
  LAS_LDWVibrationWarning/8(output8) -> or8/6
  LAS_SLASpdLimit/1(output1) -> or1/7
  LAS_SLASpdLimit/2(output2) -> or2/7
  LAS_SLASpdLimit/3(output3) -> or3/7
  LAS_SLASpdLimit/4(output4) -> or4/7
  LAS_SLASpdLimit/5(output5) -> or5/7
  LAS_SLASpdLimit/6(output6) -> or6/7
  LAS_SLASpdLimit/7(output7) -> or7/7
  LAS_SLASpdLimit/8(output8) -> or8/7
  LAS_LDWReminder/1(output1) -> or1/8
  LAS_LDWReminder/2(output2) -> or2/8
  LAS_LDWReminder/3(output3) -> or3/8
  LAS_LDWReminder/4(output4) -> or4/8
  LAS_LDWReminder/5(output5) -> or5/8
  LAS_LDWReminder/6(output6) -> or6/8
  LAS_LDWReminder/7(output7) -> or7/8
  LAS_LDWReminder/8(output8) -> or8/8
  LAS_DFDWarning/1(output1) -> or1/9
  LAS_DFDWarning/2(output2) -> or2/9
  LAS_DFDWarning/3(output3) -> or3/9
  LAS_DFDWarning/4(output4) -> or4/9
  LAS_DFDWarning/5(output5) -> or5/9
  LAS_DFDWarning/6(output6) -> or6/9
  LAS_DFDWarning/7(output7) -> or7/9
  LAS_DFDWarning/8(output8) -> or8/9
  LAS_LASFailed/1(output1) -> or1/10
  LAS_LASFailed/2(output2) -> or2/10
  LAS_LASFailed/3(output3) -> or3/10
  LAS_LASFailed/4(output4) -> or4/10
  LAS_LASFailed/5(output5) -> or5/10
  LAS_LASFailed/6(output6) -> or6/10
  LAS_LASFailed/7(output7) -> or7/10
  LAS_LASFailed/8(output8) -> or8/10
  LAS_SteeringTorqueReq/1(output1) -> or1/11
  LAS_SteeringTorqueReq/2(output2) -> or2/11
  LAS_SteeringTorqueReq/3(output3) -> or3/11
  LAS_SteeringTorqueReq/4(output4) -> or4/11
  LAS_SteeringTorqueReq/5(output5) -> or5/11
  LAS_SteeringTorqueReq/6(output6) -> or6/11
  LAS_SteeringTorqueReq/7(output7) -> or7/11
  LAS_SteeringTorqueReq/8(output8) -> or8/11
  LAS_SLAState/1(output1) -> or1/12
  LAS_SLAState/2(output2) -> or2/12
  LAS_SLAState/3(output3) -> or3/12
  LAS_SLAState/4(output4) -> or4/12
  LAS_SLAState/5(output5) -> or5/12
  LAS_SLAState/6(output6) -> or6/12
  LAS_SLAState/7(output7) -> or7/12
  LAS_SLAState/8(output8) -> or8/12
  LAS_LKSStatus/1(output1) -> or1/13
  LAS_LKSStatus/2(output2) -> or2/13
  LAS_LKSStatus/3(output3) -> or3/13
  LAS_LKSStatus/4(output4) -> or4/13
  LAS_LKSStatus/5(output5) -> or5/13
  LAS_LKSStatus/6(output6) -> or6/13
  LAS_LKSStatus/7(output7) -> or7/13
  LAS_LKSStatus/8(output8) -> or8/13
  RollingConter/1(output1) -> or1/14
  RollingConter/2(output2) -> or2/14
  RollingConter/3(output3) -> or3/14
  RollingConter/4(output4) -> or4/14
  RollingConter/5(output5) -> or5/14
  RollingConter/6(output6) -> or6/14
  RollingConter/7(output7) -> or7/14
  RollingConter/8(output8) -> or8/14
  CRC/1(output1) -> or1/15
  CRC/2(output2) -> or2/15
  CRC/3(output3) -> or3/15
  CRC/4(output4) -> or4/15
  CRC/5(output5) -> or5/15
  CRC/6(output6) -> or6/15
  CRC/7(output7) -> or7/15
  CRC/8(output8) -> or8/15
  or1/1 -> Conv1/1
  Conv1/1 -> LAS_28D_mux/1
  or2/1 -> Conv2/1
  Conv2/1 -> LAS_28D_mux/2
  or3/1 -> Conv3/1
  Conv3/1 -> LAS_28D_mux/3
  or4/1 -> Conv4/1
  Conv4/1 -> LAS_28D_mux/4
  or5/1 -> Conv5/1
  Conv5/1 -> LAS_28D_mux/5
  or6/1 -> Conv6/1
  Conv6/1 -> LAS_28D_mux/6
  or7/1 -> Conv7/1
  Conv7/1 -> LAS_28D_mux/7
  or8/1 -> Conv8/1
  Conv8/1 -> LAS_28D_mux/8
  LAS_28D_ID/1 -> LAS_28D_ID_Out/1
  LAS_28D_DLC/1 -> LAS_28D_DLC_Out/1
  LAS_SLASpdLimitUnit_in/1 -> LAS_SLASpdLimitUnit/1(LAS_SLASpdLimitUnit)
  LAS_LDWStatus_in/1 -> LAS_LDWStatus/1(LAS_LDWStatus)
  LAS_CaliStatus_in/1 -> LAS_CaliStatus/1(LAS_CaliStatus)
  LAS_TakeoverReq_in/1 -> LAS_TakeoverReq/1(LAS_TakeoverReq)
  LAS_DFDFailed_in/1 -> LAS_DFDFailed/1(LAS_DFDFailed)
  LAS_LDWVibrationWarning_in/1 -> LAS_LDWVibrationWarning/1(LAS_LDWVibrationWarning)
  LAS_SLASpdLimit_in/1 -> LAS_SLASpdLimit/1(LAS_SLASpdLimit)
  LAS_LDWReminder_in/1 -> LAS_LDWReminder/1(LAS_LDWReminder)
  LAS_DFDWarning_in/1 -> LAS_DFDWarning/1(LAS_DFDWarning)
  LAS_LASFailed_in/1 -> LAS_LASFailed/1(LAS_LASFailed)
  LAS_SteeringTorqueReq_in/1 -> LAS_SteeringTorqueReq/1(LAS_SteeringTorqueReq)
  LAS_SLAState_in/1 -> LAS_SLAState/1(LAS_SLAState)
  LAS_LKSStatus_in/1 -> LAS_LKSStatus/1(LAS_LKSStatus)
  RollingConter_in/1 -> RollingConter/1(RollingConter)
  CRC_in/1 -> CRC/1(CRC)

== system VCU_CS75_12_30_test/长安CS75底盘程序，20ms一次/Output/Subsystem/2E4/ACC_2E4 ==
  ACC_CDDAxEnable_in : Inport
  ACC_DecToStop_in : Inport  Port=2
  ACC_Driveoff_Request_in : Inport  Port=3
  ACC_Mode_in : Inport  Port=4
  ACC_ACCTargetAcceleration_in : Inport  Port=5
  ACC_RollingCounter_id_in : Inport  Port=6
  ACC_CheckSum_id_in : Inport  Port=7
  ACC_2E4_DLC : Constant  Value=8  OutDataTypeStr=uint8
  ACC_2E4_DLC_Out : Terminator
  ACC_2E4_ID : Constant  Value=740  OutDataTypeStr=single
  ACC_2E4_ID_Out : Terminator
  ACC_2E4_mux : Mux  Inputs=8
  ACC_ACCTargetAcceleration : Subsystem
  ACC_CDDAxEnable : Subsystem
  ACC_CheckSum_id : Subsystem
  ACC_DecToStop : Subsystem
  ACC_Driveoff_Request : Subsystem
  ACC_Mode : Subsystem
  ACC_RollingCounter_id : Subsystem
  Conv{1..8} (8 alike) : DataTypeConversion
  or{1..8} (8 alike) : simulink/Logic and Bit Operations/Bitwise Operator  logicop=OR  UseBitMask=off  NumInputPorts=7  BitMask=bin2dec('11011001')  BitMaskRealWorld=Stored Integer
  output : Outport
  wires:
  ACC_2E4_mux/1 -> output/1
  ACC_CDDAxEnable/1(output1) -> or1/1
  ACC_CDDAxEnable/2(output2) -> or2/1
  ACC_CDDAxEnable/3(output3) -> or3/1
  ACC_CDDAxEnable/4(output4) -> or4/1
  ACC_CDDAxEnable/5(output5) -> or5/1
  ACC_CDDAxEnable/6(output6) -> or6/1
  ACC_CDDAxEnable/7(output7) -> or7/1
  ACC_CDDAxEnable/8(output8) -> or8/1
  ACC_DecToStop/1(output1) -> or1/2
  ACC_DecToStop/2(output2) -> or2/2
  ACC_DecToStop/3(output3) -> or3/2
  ACC_DecToStop/4(output4) -> or4/2
  ACC_DecToStop/5(output5) -> or5/2
  ACC_DecToStop/6(output6) -> or6/2
  ACC_DecToStop/7(output7) -> or7/2
  ACC_DecToStop/8(output8) -> or8/2
  ACC_Driveoff_Request/1(output1) -> or1/3
  ACC_Driveoff_Request/2(output2) -> or2/3
  ACC_Driveoff_Request/3(output3) -> or3/3
  ACC_Driveoff_Request/4(output4) -> or4/3
  ACC_Driveoff_Request/5(output5) -> or5/3
  ACC_Driveoff_Request/6(output6) -> or6/3
  ACC_Driveoff_Request/7(output7) -> or7/3
  ACC_Driveoff_Request/8(output8) -> or8/3
  ACC_Mode/1(output1) -> or1/4
  ACC_Mode/2(output2) -> or2/4
  ACC_Mode/3(output3) -> or3/4
  ACC_Mode/4(output4) -> or4/4
  ACC_Mode/5(output5) -> or5/4
  ACC_Mode/6(output6) -> or6/4
  ACC_Mode/7(output7) -> or7/4
  ACC_Mode/8(output8) -> or8/4
  ACC_ACCTargetAcceleration/1(output1) -> or1/5
  ACC_ACCTargetAcceleration/2(output2) -> or2/5
  ACC_ACCTargetAcceleration/3(output3) -> or3/5
  ACC_ACCTargetAcceleration/4(output4) -> or4/5
  ACC_ACCTargetAcceleration/5(output5) -> or5/5
  ACC_ACCTargetAcceleration/6(output6) -> or6/5
  ACC_ACCTargetAcceleration/7(output7) -> or7/5
  ACC_ACCTargetAcceleration/8(output8) -> or8/5
  ACC_RollingCounter_id/1(output1) -> or1/6
  ACC_RollingCounter_id/2(output2) -> or2/6
  ACC_RollingCounter_id/3(output3) -> or3/6
  ACC_RollingCounter_id/4(output4) -> or4/6
  ACC_RollingCounter_id/5(output5) -> or5/6
  ACC_RollingCounter_id/6(output6) -> or6/6
  ACC_RollingCounter_id/7(output7) -> or7/6
  ACC_RollingCounter_id/8(output8) -> or8/6
  ACC_CheckSum_id/1(output1) -> or1/7
  ACC_CheckSum_id/2(output2) -> or2/7
  ACC_CheckSum_id/3(output3) -> or3/7
  ACC_CheckSum_id/4(output4) -> or4/7
  ACC_CheckSum_id/5(output5) -> or5/7
  ACC_CheckSum_id/6(output6) -> or6/7
  ACC_CheckSum_id/7(output7) -> or7/7
  ACC_CheckSum_id/8(output8) -> or8/7
  or1/1 -> Conv1/1
  Conv1/1 -> ACC_2E4_mux/1
  or2/1 -> Conv2/1
  Conv2/1 -> ACC_2E4_mux/2
  or3/1 -> Conv3/1
  Conv3/1 -> ACC_2E4_mux/3
  or4/1 -> Conv4/1
  Conv4/1 -> ACC_2E4_mux/4
  or5/1 -> Conv5/1
  Conv5/1 -> ACC_2E4_mux/5
  or6/1 -> Conv6/1
  Conv6/1 -> ACC_2E4_mux/6
  or7/1 -> Conv7/1
  Conv7/1 -> ACC_2E4_mux/7
  or8/1 -> Conv8/1
  Conv8/1 -> ACC_2E4_mux/8
  ACC_2E4_ID/1 -> ACC_2E4_ID_Out/1
  ACC_2E4_DLC/1 -> ACC_2E4_DLC_Out/1
  ACC_CDDAxEnable_in/1 -> ACC_CDDAxEnable/1(ACC_CDDAxEnable)
  ACC_DecToStop_in/1 -> ACC_DecToStop/1(ACC_DecToStop)
  ACC_Driveoff_Request_in/1 -> ACC_Driveoff_Request/1(ACC_Driveoff_Request)
  ACC_Mode_in/1 -> ACC_Mode/1(ACC_Mode)
  ACC_ACCTargetAcceleration_in/1 -> ACC_ACCTargetAcceleration/1(ACC_ACCTargetAcceleration)
  ACC_RollingCounter_id_in/1 -> ACC_RollingCounter_id/1(ACC_RollingCounter_id)
  ACC_CheckSum_id_in/1 -> ACC_CheckSum_id/1(ACC_CheckSum_id)
